simulink model "test14_r2019b"  (R2022b)
settings: Solver=VariableStepAuto  StartTime=0.0  StopTime=20  FixedStep=0.001  MaxStep=0.1  RelTol=1e-3
model workspace: external: MATLAB File E:\Hoc\do an\(final) download\test14_DataFile.m (data not in the file)
undefined symbols (not defined in the file): h, km, m, s, smiData, X, Y, Z
libraries: sm_lib x318, aerolibconvert2 x31, simulink_extras x25, nesl_utility x22, autolibshared x6, slpidlib x2, vehdynlibsteering x1
(part 1 of 9)
settings Model: Creator=ASUS  LastModifiedBy=ASUS
settings SolverCC: ZeroCrossAlgorithm=Adaptive  AlgebraicLoopSolver=LineSearch
settings DebuggingCC: IgnoredZcDiagnostic=none

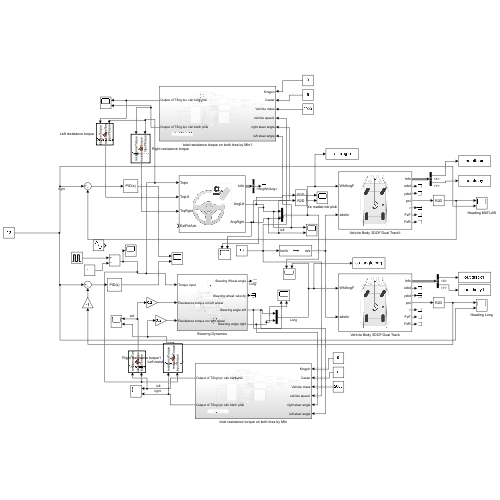
[thumbnail: Simulink's stored preview of the top-level diagram]
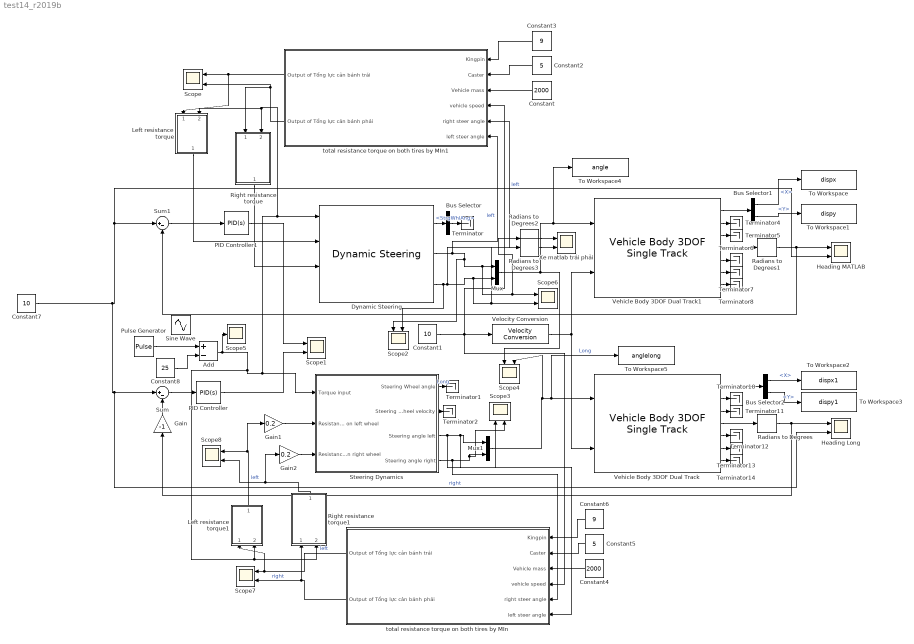
== system test14_r2019b ==
  Add : Sum  Inputs=+-
  Bus Selector : BusSelector  OutputSignals=StrgWhlAng
  Bus Selector1 : BusSelector  OutputSignals=InertFrm.Cg.Disp.X,InertFrm.Cg.Disp.Y
  Bus Selector2 : BusSelector  OutputSignals=InertFrm.Cg.Disp.X,InertFrm.Cg.Disp.Y
  Constant : Constant  Value=2000
  Constant1 : Constant  Value=10
  Constant2 : Constant  Value=5
  Constant3 : Constant  Value=9
  Constant4 : Constant  Value=2000
  Constant5 : Constant  Value=5
  Constant6 : Constant  Value=9
  Constant7 : Constant  Value=10
  Constant8 : Constant  Value=25
  Dynamic Steering : vehdynlibsteering/Dynamic Steering  StrgType=Rack and pinion  StrgRatioType=Constant  PwrAst=off  Loc=Front  TrckWdth=1  WhlBase=1.524  StrgRng=1.75*pi  StrgAngBpts="[-6.2832   -5.0265   -3.7699   -2.5133   -1.2566         0    1.2566    2.5133    3.7699    5.0265    6.2832]"  StrgRatioTbl=|  StrgRatio=13.5  StrgArmLngth=0.1  RckCsLngth=0.5  TieRodLngth=0.248  D=0.2  PnnRadiusTbl="[0.0055    0.0055    0.0056    0.0057    0.0057    0.0057    0.0058    0.0057    0.0056    0.0055    0.0055]"  PnnRadius=0.0057  RodLngth=0.1  ParaArmLngth=0.9  J1=0.1  J2=0.01  beta_u=0.1  beta_l=0.1  b1=0.001  k1=30  b2=1  b3=0.001  theta_o=0  omega_o=0  FricTrq=0  TrqBpts=[-100 0 100]  VehSpdBpts=[0 20]  TrqTbl=[0 -100;0 0;0 100]  TrqLmt=100  PwrLmt=1000  Eta=1  omega_c=200  aMode=2
      | [13.5000   13.3750   13.2500   13.1250   13.0000   13.0000   13.0000   13.1250   13.2500   13.3750   13.5000
      | ]
  Gain : Gain  Gain=-1
  Gain1 : Gain  Gain=0.2
  Gain2 : Gain  Gain=0.2
  Heading Long : Scope  NumInputPorts=2
  Heading MATLAB : Scope  NumInputPorts=2
  Left resistance torque : MATLAB Function  TreatAsAtomicUnit=on
  Left resistance torque1 : MATLAB Function  TreatAsAtomicUnit=on
  Mux : Mux  Inputs=2
  Mux1 : Mux  Inputs=2
  PID Controller : slpidlib/PID Controller  Controller=PID  Form=Parallel  TimeDomain=Continuous-time  UseExternalTs=off  SampleTime=-1  IntegratorMethod=Forward Euler  FilterMethod=Forward Euler  ControllerParametersSource=internal  P=1  I=1  UseKiTs=off  D=1  N=100  UseFilter=on  TunerSelectOption=Transfer Function Based (PID Tuner App)  InitialConditionSource=internal  InitialConditionForIntegrator=0  InitialConditionForFilter=0  DifferentiatorICPrevScaledInput=0  ExternalReset=none  TrackingMode=off  Kt=1  LimitOutput=off  SatLimitsSource=internal  UpperSaturationLimit=inf  LowerSaturationLimit=-inf  LinearizeAsGain=on  AntiWindupMode=none  Kb=1  LimitIntegrator=off  UpperIntegratorSaturationLimit=inf  LowerIntegratorSaturationLimit=-inf  POutMin=[]  POutMax=[]  IOutMin=[]  IOutMax=[]  DOutMin=[]  DOutMax=[]  NOutMin=[]  NOutMax=[]  SumOutMin=[]  SumOutMax=[]  SaturationOutMin=[]  SaturationOutMax=[]  PParamMin=[]  PParamMax=[]  IParamMin=[]  IParamMax=[]  DParamMin=[]  DParamMax=[]  NParamMin=[]  NParamMax=[]  KbParamMin=[]  KbParamMax=[]  KtParamMin=[]  KtParamMax=[]  KbOutMin=[]  KbOutMax=[]  KtOutMin=[]  KtOutMax=[]  IntegratorOutMin=[]  IntegratorOutMax=[]  FilterOutMin=[]  FilterOutMax=[]  SumI1OutMin=[]  SumI1OutMax=[]  SumI2OutMin=[]  SumI2OutMax=[]  SumI3OutMin=[]  SumI3OutMax=[]  SumI4OutMin=[]  SumI4OutMax=[]  SumDOutMin=[]  SumDOutMax=[]  DifferentiatorOutMin=[]  DifferentiatorOutMax=[]  FilterDiffOutCoefMin=[]  FilterDiffOutCoefMax=[]  ReciprocalOutMin=[]  ReciprocalOutMax=[]  SumDenOutMin=[]  SumDenOutMax=[]  SumNumOutMin=[]  SumNumOutMax=[]  DivideOutMin=[]  DivideOutMax=[]  UdiffTsProdOutMin=[]  UdiffTsProdOutMax=[]  NTsProdOutMin=[]  NTsProdOutMax=[]  UintegralTsProdOutMin=[]  UintegralTsProdOutMax=[]  UngainTsProdOutMin=[]  UngainTsProdOutMax=[]  ClampingZeroOutDataTypeStr=Inherit: Inherit via back propagation  ClampingZeroOutMin=[]  ClampingZeroOutMax=[]  FilterDenConstantOutDataTypeStr=Inherit: Inherit via back propagation  FilterDenConstantOutMin=[]  FilterDenConstantOutMax=[]  PCopyOutDataTypeStr=Inherit: Inherit via back propagation  PCopyOutMin=[]  PCopyOutMax=[]  NCopyOutDataTypeStr=Inherit: Inherit via back propagation  NCopyOutMin=[]  NCopyOutMax=[]  IntegratorContinuousStateAttributes=''  IntegratorStateMustResolveToSignalObject=off  IntegratorRTWStateStorageClass=Auto  FilterContinuousStateAttributes=''  FilterStateMustResolveToSignalObject=off  FilterRTWStateStorageClass=Auto  ParallelPVariant=InternalParameters  IdealPVariant=Disabled  IVariant=InternalParameters  DVariant=InternalParameters  IntegratorVariant=Continuous  SatVariant=Disabled  AWVariant=Passthrough  PCopyVariant=Disabled  TRVariant=Disabled  FdbkBlocksVariant=Forward  IdealPFdbkVariant=Disabled  SatFdbkVariant=Disabled  DerivativeFilterVariant=ContFilter  NVariant=InternalParameters  NCopyVariant=Disabled  FilterICVariant=InternalICsFilter  IntegratorICVariant=InternalICs  ExternalResetVariant=Disabled  TRSumVariant=Passthrough  SumFdbkVariant=Disabled  SumVariant=Sum_PID  TsampFilterVariant=InternalTs  TsampNgainVariant=Passthrough  TsampIntegralVariant=Passthrough  ExternalSaturationOutDataTypeStr=Inherit: Same as second input
  PID Controller1 : slpidlib/PID Controller  Controller=PID  Form=Parallel  TimeDomain=Continuous-time  UseExternalTs=off  SampleTime=-1  IntegratorMethod=Forward Euler  FilterMethod=Forward Euler  ControllerParametersSource=internal  P=1  I=1  UseKiTs=off  D=1  N=100  UseFilter=on  TunerSelectOption=Transfer Function Based (PID Tuner App)  InitialConditionSource=internal  InitialConditionForIntegrator=0  InitialConditionForFilter=0  DifferentiatorICPrevScaledInput=0  ExternalReset=none  TrackingMode=off  Kt=1  LimitOutput=off  SatLimitsSource=internal  UpperSaturationLimit=inf  LowerSaturationLimit=-inf  LinearizeAsGain=on  AntiWindupMode=none  Kb=1  LimitIntegrator=off  UpperIntegratorSaturationLimit=inf  LowerIntegratorSaturationLimit=-inf  POutMin=[]  POutMax=[]  IOutMin=[]  IOutMax=[]  DOutMin=[]  DOutMax=[]  NOutMin=[]  NOutMax=[]  SumOutMin=[]  SumOutMax=[]  SaturationOutMin=[]  SaturationOutMax=[]  PParamMin=[]  PParamMax=[]  IParamMin=[]  IParamMax=[]  DParamMin=[]  DParamMax=[]  NParamMin=[]  NParamMax=[]  KbParamMin=[]  KbParamMax=[]  KtParamMin=[]  KtParamMax=[]  KbOutMin=[]  KbOutMax=[]  KtOutMin=[]  KtOutMax=[]  IntegratorOutMin=[]  IntegratorOutMax=[]  FilterOutMin=[]  FilterOutMax=[]  SumI1OutMin=[]  SumI1OutMax=[]  SumI2OutMin=[]  SumI2OutMax=[]  SumI3OutMin=[]  SumI3OutMax=[]  SumI4OutMin=[]  SumI4OutMax=[]  SumDOutMin=[]  SumDOutMax=[]  DifferentiatorOutMin=[]  DifferentiatorOutMax=[]  FilterDiffOutCoefMin=[]  FilterDiffOutCoefMax=[]  ReciprocalOutMin=[]  ReciprocalOutMax=[]  SumDenOutMin=[]  SumDenOutMax=[]  SumNumOutMin=[]  SumNumOutMax=[]  DivideOutMin=[]  DivideOutMax=[]  UdiffTsProdOutMin=[]  UdiffTsProdOutMax=[]  NTsProdOutMin=[]  NTsProdOutMax=[]  UintegralTsProdOutMin=[]  UintegralTsProdOutMax=[]  UngainTsProdOutMin=[]  UngainTsProdOutMax=[]  ClampingZeroOutDataTypeStr=Inherit: Inherit via back propagation  ClampingZeroOutMin=[]  ClampingZeroOutMax=[]  FilterDenConstantOutDataTypeStr=Inherit: Inherit via back propagation  FilterDenConstantOutMin=[]  FilterDenConstantOutMax=[]  PCopyOutDataTypeStr=Inherit: Inherit via back propagation  PCopyOutMin=[]  PCopyOutMax=[]  NCopyOutDataTypeStr=Inherit: Inherit via back propagation  NCopyOutMin=[]  NCopyOutMax=[]  IntegratorContinuousStateAttributes=''  IntegratorStateMustResolveToSignalObject=off  IntegratorRTWStateStorageClass=Auto  FilterContinuousStateAttributes=''  FilterStateMustResolveToSignalObject=off  FilterRTWStateStorageClass=Auto  ParallelPVariant=InternalParameters  IdealPVariant=Disabled  IVariant=InternalParameters  DVariant=InternalParameters  IntegratorVariant=Continuous  SatVariant=Disabled  AWVariant=Passthrough  PCopyVariant=Disabled  TRVariant=Disabled  FdbkBlocksVariant=Forward  IdealPFdbkVariant=Disabled  SatFdbkVariant=Disabled  DerivativeFilterVariant=ContFilter  NVariant=InternalParameters  NCopyVariant=Disabled  FilterICVariant=InternalICsFilter  IntegratorICVariant=InternalICs  ExternalResetVariant=Disabled  TRSumVariant=Passthrough  SumFdbkVariant=Disabled  SumVariant=Sum_PID  TsampFilterVariant=InternalTs  TsampNgainVariant=Passthrough  TsampIntegralVariant=Passthrough  ExternalSaturationOutDataTypeStr=Inherit: Same as second input
  Pulse Generator : DiscretePulseGenerator  PulseType=Time based  Amplitude=50  Period=10  PulseWidth=50
  Radians to Degrees{,1..3} (4 alike) : simulink_extras/Transformations/Radians to Degrees
  Right resistance torque : MATLAB Function  TreatAsAtomicUnit=on
  Right resistance torque1 : MATLAB Function  TreatAsAtomicUnit=on
  Scope{,1..4,6..8} (8 alike) : Scope  NumInputPorts=2
  Scope5 : Scope
  Sine Wave : Sin  Amplitude=80  Frequency=3  SampleTime=0
  Steering Dynamics : Subsystem
  Sum : Sum  Inputs=|+-
  Sum1 : Sum  Inputs=|+-
  Terminator{,1..2,4..8,10..14} (13 alike) : Terminator
  To Workspace : ToWorkspace  VariableName=dispx  SaveFormat=Structure With Time  SampleTime=-1
  To Workspace1 : ToWorkspace  VariableName=dispy  SaveFormat=Structure With Time  SampleTime=-1
  To Workspace2 : ToWorkspace  VariableName=dispx1  SaveFormat=Structure With Time  SampleTime=-1
  To Workspace3 : ToWorkspace  VariableName=dispy1  SaveFormat=Structure With Time  SampleTime=-1
  To Workspace4 : ToWorkspace  VariableName=angle  SaveFormat=Structure With Time  SampleTime=-1
  To Workspace5 : ToWorkspace  VariableName=anglelong  SaveFormat=Structure With Time  SampleTime=-1
  Vehicle Body 3DOF Dual Track : autolibshared/Vehicle Body 3DOF Single Track  trackMode=Dual  inputMode=External longitudinal velocity  frontSteerMode=on  rearSteerMode=off  windMode=off  muMode=off  extFMode=off  extMMode=off  htchFMode=off  htchMMode=off  extXo=off  extpsio=off  extxdoto=off  extro=off  extYo=off  extTamb=off  extydoto=off  aMode=2  NF=2  NR=2  m=2000  a=1.4  b=1.6  h=0.35  dh=1  hh=0.2  X_o=0  xdot_o=0  CalphaMode=off  sigmaMode=on  d=0  hl=0  w=[1.4,1.4]  Cy_f=12e3  Cy_r=11e3  sigma_f=.1  sigma_r=.1  alpha_f_brk=[-.1 .1]  Cy_f_data=[-9e3 9e3]  alpha_r_brk=[-.1 .1]  Cy_r_data=[-9e3 9e3]  Y_o=0  ydot_o=0  Izz=4000  psi_o=0  r_o=0  Af=2  Cd=.3  Cl=.1  Cpm=.1  beta_w=[0:0.01:0.3]  Cs=[0:0.03:0.9]  Cym=[0:0.01:0.3]  Pabs=101325  Tair=273  g=9.81  mu=1  xdot_tol=.01  Fznom=5000  Fxtire_sat=7e4  Fytire_sat=7e4  longOff=0  latOff=0  vertOff=0  wrapAng=off
  Vehicle Body 3DOF Dual Track1 : autolibshared/Vehicle Body 3DOF Single Track  trackMode=Dual  inputMode=External longitudinal velocity  frontSteerMode=on  rearSteerMode=off  windMode=off  muMode=off  extFMode=off  extMMode=off  htchFMode=off  htchMMode=off  extXo=off  extpsio=off  extxdoto=off  extro=off  extYo=off  extTamb=off  extydoto=off  aMode=2  NF=2  NR=2  m=2000  a=1.4  b=1.6  h=0.35  dh=1  hh=0.2  X_o=0  xdot_o=0  CalphaMode=off  sigmaMode=on  d=0  hl=0  w=[1.4,1.4]  Cy_f=12e3  Cy_r=11e3  sigma_f=.1  sigma_r=.1  alpha_f_brk=[-.1 .1]  Cy_f_data=[-9e3 9e3]  alpha_r_brk=[-.1 .1]  Cy_r_data=[-9e3 9e3]  Y_o=0  ydot_o=0  Izz=4000  psi_o=0  r_o=0  Af=2  Cd=.3  Cl=.1  Cpm=.1  beta_w=[0:0.01:0.3]  Cs=[0:0.03:0.9]  Cym=[0:0.01:0.3]  Pabs=101325  Tair=273  g=9.81  mu=1  xdot_tol=.01  Fznom=5000  Fxtire_sat=7e4  Fytire_sat=7e4  longOff=0  latOff=0  vertOff=0  wrapAng=off
  Velocity Conversion : aerolibconvert2/Velocity Conversion  IU=km/h  OU=m/s
  Xe matlab trái phải : Scope  NumInputPorts=2
  total resistance torque on both tires by MIn : Subsystem
  total resistance torque on both tires by MIn1 : Subsystem
  wires:
  Dynamic Steering/2 -> total resistance torque on both tires by MIn1/6(left steer angle), Scope2/1, Radians to Degrees2/1, Scope6/1, Mux/1  "left"
  Dynamic Steering/3 -> Scope2/2, total resistance torque on both tires by MIn1/5(right steer angle), Radians to Degrees3/1, Scope6/2, Mux/2  "left"
  Steering Dynamics/3(Steering angle left) -> Scope3/1, total resistance torque on both tires by MIn/6(left steer angle), Mux1/1
  Steering Dynamics/4(Steering angle right) -> total resistance torque on both tires by MIn/5(right steer angle), Scope3/2, Mux1/2
  Mux1/1 -> Vehicle Body 3DOF Dual Track/1, To Workspace5/1, Scope4/2  "Long"
  Velocity Conversion/1 -> Vehicle Body 3DOF Dual Track/2, Vehicle Body 3DOF Dual Track1/2
  Constant1/1 -> total resistance torque on both tires by MIn1/4("vehicle speed "), total resistance torque on both tires by MIn/4("vehicle speed "), Velocity Conversion/1
  Vehicle Body 3DOF Dual Track1/4 -> Radians to Degrees1/1
  Vehicle Body 3DOF Dual Track/4 -> Radians to Degrees/1
  Radians to Degrees/1 -> Heading Long/1, Gain/1
  Steering Dynamics/2(Steering wheel velocity) -> Terminator2/1
  Vehicle Body 3DOF Dual Track1/1 -> Bus Selector1/1
  Vehicle Body 3DOF Dual Track1/2 -> Terminator4/1
  Vehicle Body 3DOF Dual Track1/3 -> Terminator5/1
  Vehicle Body 3DOF Dual Track1/5 -> Terminator6/1
  Vehicle Body 3DOF Dual Track1/6 -> Terminator7/1
  Vehicle Body 3DOF Dual Track1/7 -> Terminator8/1
  Vehicle Body 3DOF Dual Track/2 -> Terminator10/1
  Vehicle Body 3DOF Dual Track/3 -> Terminator11/1
  Vehicle Body 3DOF Dual Track/5 -> Terminator12/1
  Vehicle Body 3DOF Dual Track/6 -> Terminator13/1
  Vehicle Body 3DOF Dual Track/7 -> Terminator14/1
  Dynamic Steering/1 -> Bus Selector/1
  Bus Selector/1 -> Terminator/1  "<StrgWhlAng>"
  Bus Selector1/1 -> To Workspace/1  "<X>"
  Bus Selector1/2 -> To Workspace1/1  "<Y>"
  total resistance torque on both tires by MIn1/2(Output of Tổng lực cản bánh phải) -> Scope/2, Right resistance torque/1("resistanceTorque ")
  Constant/1 -> total resistance torque on both tires by MIn1/3(Vehicle mass)
  Constant2/1 -> total resistance torque on both tires by MIn1/2(Caster)
  Constant3/1 -> total resistance torque on both tires by MIn1/1(Kingpin)
  Constant4/1 -> total resistance torque on both tires by MIn/3(Vehicle mass)
  Constant5/1 -> total resistance torque on both tires by MIn/2(Caster)
  Constant6/1 -> total resistance torque on both tires by MIn/1(Kingpin)
  Vehicle Body 3DOF Dual Track/1 -> Bus Selector2/1
  Bus Selector2/1 -> To Workspace2/1  "<X>"
  Bus Selector2/2 -> To Workspace3/1  "<Y>"
  Steering Dynamics/1(Steering Wheel angle) -> Terminator1/1  "Long"
  Sum/1 -> PID Controller/1
  Sum1/1 -> PID Controller1/1
  PID Controller1/1 -> Scope1/1
  Radians to Degrees1/1 -> Sum1/2, Heading MATLAB/1
  PID Controller/1 -> Scope1/2
  Constant7/1 -> Heading Long/2, Sum/1, Heading MATLAB/2, Sum1/1  "right"
  Gain/1 -> Sum/2
  Mux/1 -> Scope4/1, To Workspace4/1, Vehicle Body 3DOF Dual Track1/1
  Pulse Generator/1 -> Add/1
  Constant8/1 -> Add/2
  total resistance torque on both tires by MIn/1(Output of Tổng lực cản bánh trái) -> Left resistance torque1/1("resistanceTorque "), Scope7/1  "left"
  total resistance torque on both tires by MIn/2(Output of Tổng lực cản bánh phải) -> Scope7/2, Right resistance torque1/1("resistanceTorque ")  "right"
  total resistance torque on both tires by MIn1/1(Output of Tổng lực cản bánh trái) -> Left resistance torque/1("resistanceTorque "), Scope/1
  Add/1 -> Scope5/1, Right resistance torque1/2(inputTorque), Left resistance torque1/2(inputTorque), Left resistance torque/2(inputTorque), Right resistance torque/2(inputTorque), Dynamic Steering/1, Steering Dynamics/1(Torque input)
  Left resistance torque1/1(resistanceTorque) -> Gain1/1, Scope8/1  "left"
  Radians to Degrees2/1 -> Xe matlab trái phải/1
  Radians to Degrees3/1 -> Xe matlab trái phải/2
  Right resistance torque1/1(resistanceTorque) -> Gain2/1, Scope8/2
  Right resistance torque/1(resistanceTorque) -> Dynamic Steering/3
  Left resistance torque/1(resistanceTorque) -> Dynamic Steering/2
  Gain1/1 -> Steering Dynamics/2(Resistance torque on left wheel)
  Gain2/1 -> Steering Dynamics/3(Resistance torque on right wheel)

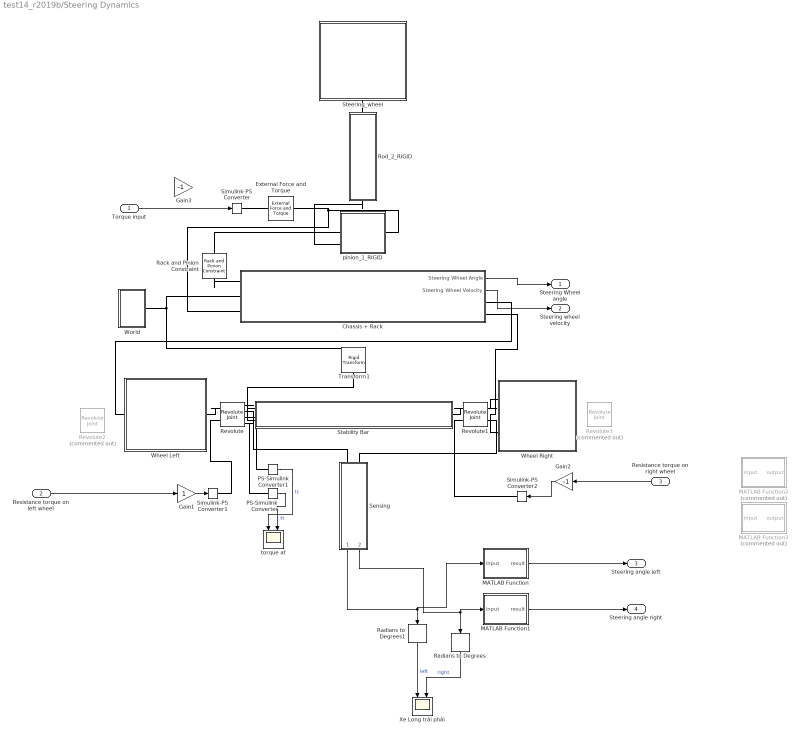
== system test14_r2019b/Steering Dynamics ==
  Torque input : Inport
  Resistance torque on left wheel : Inport  Port=2
  Resistance torque on right wheel : Inport  Port=3
  Chassis + Rack : Subsystem
      mask Display: image('$imagefile'); % Use "Edit Image" on toolstrip to change.
  External Force and Torque : sm_lib/Forces and Torques/External Force and Torque  ForceResolutionFrame=AttachedFrame  EnableForceX=off  EnableForceY=off  EnableForceZ=off  EnableForce=off  TorqueResolutionFrame=AttachedFrame  EnableTorqueX=off  EnableTorqueY=off  EnableTorqueZ=on  EnableTorque=off
  Gain1 : Gain
  Gain2 : Gain  Gain=-1
  Gain3 : Gain  Gain=-1
  MATLAB Function : MATLAB Function  TreatAsAtomicUnit=on
  MATLAB Function1 : MATLAB Function  TreatAsAtomicUnit=on
  MATLAB Function2 : MATLAB Function  Commented=on  TreatAsAtomicUnit=on
  MATLAB Function3 : MATLAB Function  Commented=on  TreatAsAtomicUnit=on
  PS-Simulink Converter : nesl_utility/PS-Simulink Converter  PhysicalDomain=network_engine_domain  SubClassName=ps_output  LeftPortType=input  RightPortType=output  PseudoPeriodic=off  Frequencies=[]  VectorFormat=inherit  Unit=inherit  AffineConversion=off
  PS-Simulink Converter1 : nesl_utility/PS-Simulink Converter  PhysicalDomain=network_engine_domain  SubClassName=ps_output  LeftPortType=input  RightPortType=output  PseudoPeriodic=off  Frequencies=[]  VectorFormat=inherit  Unit=inherit  AffineConversion=off
  Rack and Pinion Constraint : sm_lib/Gears and Couplings/Gears/Rack and Pinion Constraint  PinionRadius=30  PinionRadiusUnits=mm
  Radians to Degrees : simulink_extras/Transformations/Radians to Degrees
  Radians to Degrees1 : simulink_extras/Transformations/Radians to Degrees
  Revolute : sm_lib/Joints/Revolute Joint  JointMode=Normal  SenseConstraintForce=off  SenseConstraintForceX=off  SenseConstraintForceY=off  SenseConstraintForceZ=off  SenseConstraintTorque=on  SenseConstraintTorqueX=off  SenseConstraintTorqueY=off  SenseConstraintTorqueZ=off  SenseTotalForce=off  SenseTotalForceX=off  SenseTotalForceY=off  SenseTotalForceZ=off  SenseTotalTorque=on  SenseTotalTorqueX=off  SenseTotalTorqueY=off  SenseTotalTorqueZ=off  CompositeWrenchDir=BaseOnFollower  CompositeWrenchFrame=FollowerFrame  EquilibriumPosition=0  EquilibriumPositionUnits=deg  SpringStiffness=0.0524-0.0524+0.1  SpringStiffnessUnits=N*m/deg  DampingCoefficient=1.5-1.5+0.1  DampingCoefficientUnits=N*m/(deg/s)  TorqueActuationMode=InputTorque  MotionActuationMode=ComputedMotion  SensePosition=on  SenseVelocity=off  SenseAcceleration=off  SenseTorqueForce=off  SenseLowerLimitTorqueForce=off  SenseUpperLimitTorqueForce=off  LowerLimitSpecify=on  LowerLimitBound=-89.68-28.95  LowerLimitBoundUnits=deg  LowerLimitStiffness=1e4  LowerLimitStiffnessUnits=N*m/deg  LowerLimitDamping=100  LowerLimitDampingUnits=N*m/(deg/s)  LowerLimitTransitionRegionWidth=0.1  LowerLimitTransitionRegionWidthUnits=deg  UpperLimitSpecify=on  UpperLimitBound=-89.68+18.80  UpperLimitBoundUnits=deg  UpperLimitStiffness=1e4  UpperLimitStiffnessUnits=N*m/deg  UpperLimitDamping=100  UpperLimitDampingUnits=N*m/(deg/s)  UpperLimitTransitionRegionWidth=0.1  UpperLimitTransitionRegionWidthUnits=deg  PositionTargetSpecify=on  PositionTargetPriority=High  PositionTargetValue=-89.678329494  PositionTargetValueUnits=deg  VelocityTargetSpecify=on  VelocityTargetPriority=High  VelocityTargetValue=0  VelocityTargetValueUnits=deg/s
  Revolute1 : sm_lib/Joints/Revolute Joint  JointMode=Normal  SenseConstraintForce=off  SenseConstraintForceX=off  SenseConstraintForceY=off  SenseConstraintForceZ=off  SenseConstraintTorque=off  SenseConstraintTorqueX=off  SenseConstraintTorqueY=off  SenseConstraintTorqueZ=off  SenseTotalForce=off  SenseTotalForceX=off  SenseTotalForceY=off  SenseTotalForceZ=off  SenseTotalTorque=off  SenseTotalTorqueX=off  SenseTotalTorqueY=off  SenseTotalTorqueZ=off  CompositeWrenchDir=FollowerOnBase  CompositeWrenchFrame=FollowerFrame  EquilibriumPosition=0  EquilibriumPositionUnits=deg  SpringStiffness=0.1  SpringStiffnessUnits=N*m/deg  DampingCoefficient=0.1  DampingCoefficientUnits=N*m/(deg/s)  TorqueActuationMode=InputTorque  MotionActuationMode=ComputedMotion  SensePosition=on  SenseVelocity=off  SenseAcceleration=off  SenseTorqueForce=off  SenseLowerLimitTorqueForce=off  SenseUpperLimitTorqueForce=off  LowerLimitSpecify=on  LowerLimitBound=-89.68-28.95  LowerLimitBoundUnits=deg  LowerLimitStiffness=1e4  LowerLimitStiffnessUnits=N*m/deg  LowerLimitDamping=100  LowerLimitDampingUnits=N*m/(deg/s)  LowerLimitTransitionRegionWidth=0.1  LowerLimitTransitionRegionWidthUnits=deg  UpperLimitSpecify=on  UpperLimitBound=-89.68+18.80  UpperLimitBoundUnits=deg  UpperLimitStiffness=1e4  UpperLimitStiffnessUnits=N*m/deg  UpperLimitDamping=100  UpperLimitDampingUnits=N*m/(deg/s)  UpperLimitTransitionRegionWidth=0.1  UpperLimitTransitionRegionWidthUnits=deg  PositionTargetSpecify=on  PositionTargetPriority=Low  PositionTargetValue=smiData.RevoluteJoint(2).Rz.Pos-2.7  PositionTargetValueUnits=deg  VelocityTargetSpecify=on  VelocityTargetPriority=High  VelocityTargetValue=0  VelocityTargetValueUnits=deg/s
  Revolute2 : sm_lib/Joints/Revolute Joint  Commented=on  JointMode=Normal  SenseConstraintForce=off  SenseConstraintForceX=off  SenseConstraintForceY=off  SenseConstraintForceZ=off  SenseConstraintTorque=off  SenseConstraintTorqueX=off  SenseConstraintTorqueY=off  SenseConstraintTorqueZ=off  SenseTotalForce=off  SenseTotalForceX=off  SenseTotalForceY=off  SenseTotalForceZ=off  SenseTotalTorque=off  SenseTotalTorqueX=off  SenseTotalTorqueY=off  SenseTotalTorqueZ=off  CompositeWrenchDir=BaseOnFollower  CompositeWrenchFrame=FollowerFrame  EquilibriumPosition=0  EquilibriumPositionUnits=deg  SpringStiffness=0.0524-0.0524+0.1  SpringStiffnessUnits=N*m/deg  DampingCoefficient=1.5-1.5+0.1  DampingCoefficientUnits=N*m/(deg/s)  TorqueActuationMode=InputTorque  MotionActuationMode=ComputedMotion  SensePosition=on  SenseVelocity=off  SenseAcceleration=off  SenseTorqueForce=off  SenseLowerLimitTorqueForce=off  SenseUpperLimitTorqueForce=off  LowerLimitSpecify=on  LowerLimitBound=-2+0.089+0.071  LowerLimitBoundUnits=rad  LowerLimitStiffness=1e4  LowerLimitStiffnessUnits=N*m/deg  LowerLimitDamping=100  LowerLimitDampingUnits=N*m/(deg/s)  LowerLimitTransitionRegionWidth=0.1  LowerLimitTransitionRegionWidthUnits=deg  UpperLimitSpecify=on  UpperLimitBound=-1-0.195-0.106  UpperLimitBoundUnits=rad  UpperLimitStiffness=1e4  UpperLimitStiffnessUnits=N*m/deg  UpperLimitDamping=100  UpperLimitDampingUnits=N*m/(deg/s)  UpperLimitTransitionRegionWidth=0.1  UpperLimitTransitionRegionWidthUnits=deg  PositionTargetSpecify=on  PositionTargetPriority=High  PositionTargetValue=-89.678329494  PositionTargetValueUnits=deg  VelocityTargetSpecify=on  VelocityTargetPriority=High  VelocityTargetValue=0  VelocityTargetValueUnits=deg/s
  Revolute3 : sm_lib/Joints/Revolute Joint  Commented=on  JointMode=Normal  SenseConstraintForce=off  SenseConstraintForceX=off  SenseConstraintForceY=off  SenseConstraintForceZ=off  SenseConstraintTorque=off  SenseConstraintTorqueX=off  SenseConstraintTorqueY=off  SenseConstraintTorqueZ=off  SenseTotalForce=off  SenseTotalForceX=off  SenseTotalForceY=off  SenseTotalForceZ=off  SenseTotalTorque=off  SenseTotalTorqueX=off  SenseTotalTorqueY=off  SenseTotalTorqueZ=off  CompositeWrenchDir=FollowerOnBase  CompositeWrenchFrame=FollowerFrame  EquilibriumPosition=0  EquilibriumPositionUnits=deg  SpringStiffness=0.1  SpringStiffnessUnits=N*m/deg  DampingCoefficient=0.1  DampingCoefficientUnits=N*m/(deg/s)  TorqueActuationMode=InputTorque  MotionActuationMode=ComputedMotion  SensePosition=on  SenseVelocity=off  SenseAcceleration=off  SenseTorqueForce=off  SenseLowerLimitTorqueForce=off  SenseUpperLimitTorqueForce=off  LowerLimitSpecify=off  LowerLimitBound=-2  LowerLimitBoundUnits=rad  LowerLimitStiffness=1e4  LowerLimitStiffnessUnits=N*m/deg  LowerLimitDamping=100  LowerLimitDampingUnits=N*m/(deg/s)  LowerLimitTransitionRegionWidth=0.1  LowerLimitTransitionRegionWidthUnits=deg  UpperLimitSpecify=off  UpperLimitBound=-1  UpperLimitBoundUnits=rad  UpperLimitStiffness=1e4  UpperLimitStiffnessUnits=N*m/deg  UpperLimitDamping=100  UpperLimitDampingUnits=N*m/(deg/s)  UpperLimitTransitionRegionWidth=0.1  UpperLimitTransitionRegionWidthUnits=deg  PositionTargetSpecify=on  PositionTargetPriority=Low  PositionTargetValue=smiData.RevoluteJoint(2).Rz.Pos-2.7  PositionTargetValueUnits=deg  VelocityTargetSpecify=on  VelocityTargetPriority=High  VelocityTargetValue=0  VelocityTargetValueUnits=deg/s
  Rod_2_RIGID : Subsystem
      mask Display: image('rod.png'); % Use "Edit Image" on toolstrip to change.
  "Sensing " : Subsystem
  Simulink-PS Converter : nesl_utility/Simulink-PS Converter  PhysicalDomain=network_engine_domain  SubClassName=ps_input  LeftPortType=input  RightPortType=output  PseudoPeriodic=off  Frequencies=[]  NoiseDistribution=none  NoiseParameters=[]  Unit=N*m  AffineConversion=off  FilteringAndDerivatives=provide  SimscapeFilterOrder=1  InputFilterTimeConstant=0.001  UdotUserProvided=0
  Simulink-PS Converter1 : nesl_utility/Simulink-PS Converter  PhysicalDomain=network_engine_domain  SubClassName=ps_input  LeftPortType=input  RightPortType=output  PseudoPeriodic=off  Frequencies=[]  NoiseDistribution=none  NoiseParameters=[]  Unit=N*m  AffineConversion=off  FilteringAndDerivatives=provide  SimscapeFilterOrder=1  InputFilterTimeConstant=0.001  UdotUserProvided=0
  Simulink-PS Converter2 : nesl_utility/Simulink-PS Converter  PhysicalDomain=network_engine_domain  SubClassName=ps_input  LeftPortType=input  RightPortType=output  PseudoPeriodic=off  Frequencies=[]  NoiseDistribution=none  NoiseParameters=[]  Unit=N*m  AffineConversion=off  FilteringAndDerivatives=provide  SimscapeFilterOrder=2  InputFilterTimeConstant=0.001  UdotUserProvided=0
  Stability Bar : Subsystem
      mask Display: image('$imagefile'); % Use "Edit Image" on toolstrip to change.
  Steering_wheel : Subsystem
      mask Display: image('$imagefile'); % Use "Edit Image" on toolstrip to change.
  Transform1 : sm_lib/Frames and Transforms/Rigid Transform  TranslationMethod=Cartesian  TranslationStandardOffset=0  TranslationLengthUnit=mm  TranslationStandardAxis=+Z  TranslationCartesianOffset=smiData.RigidTransform(48).translation  TranslationROffset=0  TranslationROffsetUnits=m  TranslationZOffset=0  TranslationZOffsetUnits=m  TranslationThetaOffset=0  TranslationThetaOffsetUnits=deg  RotationMethod=ArbitraryAxis  RotationAngleUnits=rad  RotationStandardAxis=+Z  RotationAngle=smiData.RigidTransform(48).angle  RotationArbitraryAxis=smiData.RigidTransform(48).axis  FollAlignAxisA=+X  BaseAlignAxisA=+Y  FollAlignAxisB=+Y  BaseAlignAxisB=+Z  RotationSequenceAxes=FollowerAxes  RotationSequence=XYX  RotationSequenceAngles=[0 0 0]  RotationSequenceAnglesUnits=deg  RotationMatrix=[1 0 0; 0 1 0; 0 0 1]  Quaternion=[1 0 0 0]
  Wheel Left : Subsystem
      mask Display: image('$imagefile'); % Use "Edit Image" on toolstrip to change.
  Wheel Right : Subsystem
      mask Display: image('$imagefile'); % Use "Edit Image" on toolstrip to change.
  World : Subsystem
  Xe Long trái phải : Scope  NumInputPorts=2
  pinion_1_RIGID : Subsystem
      mask Display: image('pinion.png'); % Use "Edit Image" on toolstrip to change.
  "torque at " : Scope  NumInputPorts=2
  Steering Wheel angle : Outport
  Steering wheel velocity : Outport  Port=2
  Steering angle left : Outport  Port=3
  Steering angle right : Outport  Port=4
  wires:
  "Sensing "/2(Steering angle right (rad)) -> MATLAB Function1/1(input), Radians to Degrees/1
  Radians to Degrees/1 -> Xe Long trái phải/2  "right"
  Radians to Degrees1/1 -> Xe Long trái phải/1  "left"
  Chassis + Rack/2(Steering Wheel Velocity) -> Steering wheel velocity/1
  Chassis + Rack/1(Steering Wheel Angle) -> Steering Wheel angle/1
  Resistance torque on left wheel/1 -> Gain1/1
  Resistance torque on right wheel/1 -> Gain2/1
  Gain1/1 -> Simulink-PS Converter1/1
  Gain2/1 -> Simulink-PS Converter2/1
  MATLAB Function/1(result) -> Steering angle left/1
  MATLAB Function1/1(result) -> Steering angle right/1
  Torque input/1 -> Simulink-PS Converter/1
  "Sensing "/1(Steering angle left (rad)) -> MATLAB Function/1(input), Radians to Degrees1/1
  PS-Simulink Converter1/1 -> "torque at "/1  "tc"
  PS-Simulink Converter/1 -> "torque at "/2  "tt"
  connections:
  Revolute/RConn2 -- "Sensing "/LConn1
  Simulink-PS Converter/RConn1 -- External Force and Torque/LConn1
  Chassis + Rack/LConn2 -- World/LConn1 -- Transform1/LConn1
  Rack and Pinion Constraint/RConn1 -- Chassis + Rack/LConn1
  Revolute1/RConn2 -- "Sensing "/LConn2
  Rack and Pinion Constraint/LConn1 -- pinion_1_RIGID/LConn2
  Transform1/RConn1 -- Stability Bar/LConn2
  Chassis + Rack/LConn3 -- pinion_1_RIGID/RConn1 -- External Force and Torque/RConn1
  Chassis + Rack/RConn1 -- Wheel Left/LConn1
  Revolute1/RConn1 -- Wheel Right/LConn1
  Chassis + Rack/RConn2 -- Wheel Right/LConn2
  Revolute1/LConn1 -- Stability Bar/RConn1
  Revolute/RConn1 -- Stability Bar/LConn1
  Revolute/LConn1 -- Wheel Left/RConn1
  Rod_2_RIGID/RConn1 -- pinion_1_RIGID/LConn3
  Steering_wheel/LConn1 -- Rod_2_RIGID/LConn1
  Simulink-PS Converter1/RConn1 -- Revolute/LConn2
  Revolute1/LConn2 -- Simulink-PS Converter2/RConn1
  Revolute/RConn3 -- PS-Simulink Converter1/LConn1
  Revolute/RConn4 -- PS-Simulink Converter/LConn1

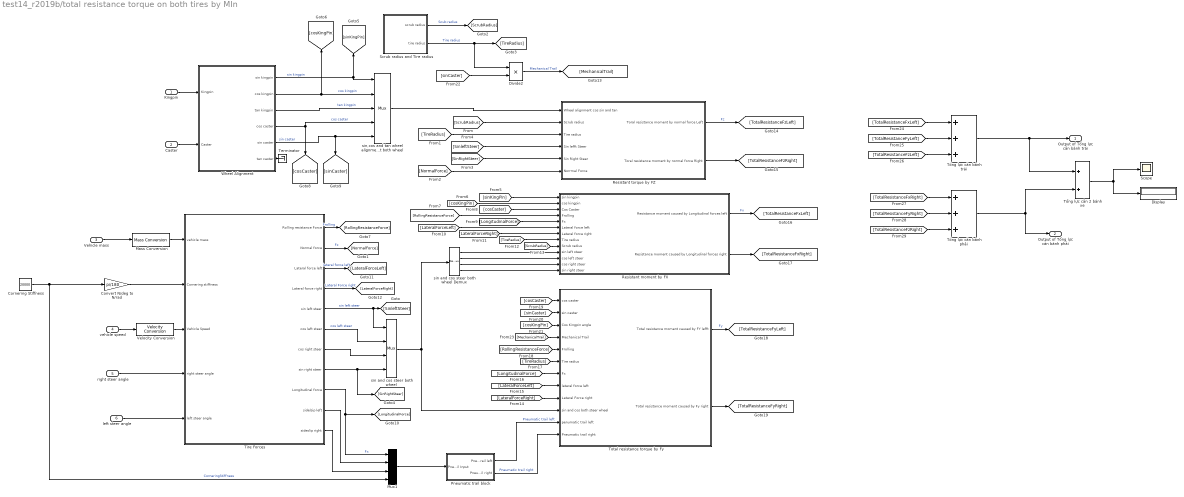
== system test14_r2019b/total resistance torque on both tires by MIn ==
  Kingpin : Inport
  Caster : Inport  Port=2
  Vehicle mass : Inport  Port=3
  "vehicle speed " : Inport  Port=4
  right steer angle : Inport  Port=5
  left steer angle : Inport  Port=6
  Convert N/deg to N/rad : Gain  Gain=pi/180
  Cornering Stiffness : Constant  Value=20000
  Display : Display
  Divide2 : Product  Inputs=**
  Mass Conversion : aerolibconvert2/Mass Conversion  IU=kg  OU=kg
  Mux1 : Mux
  Pneumatic trail block : Subsystem
  Resistant moment by FX : Subsystem
  Resistant torque by FZ : Subsystem
  Scope : Scope
  Scrub radius and Tire radius : Subsystem
  Terminator : Terminator
  Tire Forces : Subsystem
  Total resistance torque by Fy : Subsystem
  Tổng lực cản 2 bánh xe : Sum
  Tổng lực cản bánh phải : Sum  Inputs=+++
  Tổng lực cản bánh trái : Sum  Inputs=+++
  Velocity Conversion : aerolibconvert2/Velocity Conversion  IU=km/h  OU=m/s
  Wheel Alignment : Subsystem
  sin and cos steer both wheel : Mux
  sin and cos steer both wheel Demux : Demux
  sin,cos and tan wheel alignment both wheel : Mux  Inputs=5
  Output of Tổng lực cản bánh trái : Outport
  Output of Tổng lực cản bánh phải : Outport  Port=2
  wires:
  Kingpin/1 -> Wheel Alignment/1(Kingpin)
  Wheel Alignment/6(tan caster) -> Terminator/1
  Vehicle mass/1 -> Mass Conversion/1
  Mass Conversion/1 -> Tire Forces/1(vehicle mass)
  Convert N/deg to N/rad/1 -> Tire Forces/2(Cornering stiffness)
  Cornering Stiffness/1 -> Mux1/4, Convert N/deg to N/rad/1  "CorneringStiffness"
  Caster/1 -> Wheel Alignment/2(Caster)
  "vehicle speed "/1 -> Velocity Conversion/1
  right steer angle/1 -> Tire Forces/4("right steer angle ")
  left steer angle/1 -> Tire Forces/5("left steer angle ")
  Velocity Conversion/1 -> Tire Forces/3(Vehicle Speed)
  Tire Forces/11(sideslip right) -> Mux1/3
  Tire Forces/10(sidelsip left) -> Mux1/2
  Tire Forces/9(Longitudinal force) -> [LongitudinalForce], Mux1/1  "Fx"
  Mux1/1 -> Pneumatic trail block/1(Pneumatic trail Input)
  Pneumatic trail block/2(Pneumatic Trail right) -> Total resistance torque by Fy/12(Pneumatic trail right)  "Pneumatic trail right"
  Pneumatic trail block/1(Pneumatic Trail left) -> Total resistance torque by Fy/11(penumatic trail left)  "Pneumatic trail left"
  Tire Forces/5(sin left steer) -> sin and cos steer both wheel/1, [SinleftSteer]  "sin left steer"
  Tire Forces/6(cos left steer) -> sin and cos steer both wheel/2  "cos left steer"
  Tire Forces/7(cos right steer) -> sin and cos steer both wheel/3
  Tire Forces/8(sin right steer) -> [SinRightSteer], sin and cos steer both wheel/4
  sin and cos steer both wheel/1 -> sin and cos steer both wheel Demux/1, Total resistance torque by Fy/10(sin and cos both steer wheel)
  Wheel Alignment/1(sin kingpin) -> sin,cos and tan wheel alignment both wheel/1, [sinKingPin]  "sin kingpin"
  Wheel Alignment/2(cos kingpin) -> [cosKingPin], sin,cos and tan wheel alignment both wheel/2  "cos kingpin"
  Wheel Alignment/3(tan kingpin) -> sin,cos and tan wheel alignment both wheel/3  "tan kingpin"
  Wheel Alignment/4(cos caster) -> sin,cos and tan wheel alignment both wheel/4, [cosCaster]  "cos caster"
  Wheel Alignment/5(sin caster) -> [sinCaster], sin,cos and tan wheel alignment both wheel/5  "sin caster"
  sin,cos and tan wheel alignment both wheel/1 -> Resistant torque by FZ/1("Wheel alignment cos sin and tan ")
  Tire Forces/2(Normal force) -> [NormalForce]  "Fz"
  Scrub radius and Tire radius/1(scrub radius) -> [ScrubRadius]  "Scub radius"
  Scrub radius and Tire radius/2(tire radius) -> Divide2/1, [TireRadius]  "Tire radius"
  [ScrubRadius] -> Resistant torque by FZ/2(Scrub radius)
  [TireRadius] -> Resistant torque by FZ/3(Tire radius)
  [NormalForce] -> Resistant torque by FZ/6(Norrmal Force)
  [SinleftSteer] -> Resistant torque by FZ/4(Sin lefft Steer)
  [SinRightSteer] -> Resistant torque by FZ/5(Sin Right Steer)
  [sinKingPin] -> Resistant moment by FX/1(sin kingpin)
  [cosKingPin] -> Resistant moment by FX/2(cos kingpin)
  Tire Forces/1(Rolling resistance Force) -> [RollingResistanceForce]  "Frolling"
  [RollingResistanceForce] -> Resistant moment by FX/4(Frolling)
  [cosCaster] -> Resistant moment by FX/3(Cos Caster)
  [LongitudinalForce] -> Resistant moment by FX/5(Fx)
  Tire Forces/3(Lateral force left) -> [LateralForceLeft]  "lateral force left"
  Tire Forces/4(Lateral force right) -> [LateralForceRight]  "Lateral Force right"
  [LateralForceLeft] -> Resistant moment by FX/6(Lateral force left)
  [LateralForceRight] -> Resistant moment by FX/7(Lateral force right)
  [TireRadius] -> Resistant moment by FX/8(Tire radius)
  [ScrubRadius] -> Resistant moment by FX/9(Scrub radius)
  [LateralForceRight] -> Total resistance torque by Fy/9(Lateral Force right)
  [LateralForceLeft] -> Total resistance torque by Fy/8(lateral force left)
  [LongitudinalForce] -> Total resistance torque by Fy/7(Fx)
  [TireRadius] -> Total resistance torque by Fy/6(Tire radius)
  [RollingResistanceForce] -> Total resistance torque by Fy/5(Frolling)
  [sinCaster] -> Total resistance torque by Fy/2(sin caster)
  [cosCaster] -> Total resistance torque by Fy/1(cos caster)
  [cosKingPin] -> Total resistance torque by Fy/3(Cos Kingpin angle)
  sin and cos steer both wheel Demux/1 -> Resistant moment by FX/10(sin left steer)
  sin and cos steer both wheel Demux/2 -> Resistant moment by FX/11(cos left steer)
  sin and cos steer both wheel Demux/3 -> Resistant moment by FX/12(cos right steer)
  sin and cos steer both wheel Demux/4 -> Resistant moment by FX/13(sin right steer)
  [sinCaster] -> Divide2/2
  Divide2/1 -> [MechanicalTrail]  "Mechanical Trail"
  [MechanicalTrail] -> Total resistance torque by Fy/4(Mechanical Trail)
  Resistant torque by FZ/1(Toral resistance moment by normal force Left) -> [TotalResistanceFzLeft]  "Fz"
  Resistant torque by FZ/2(Toral resistance moment by normal force Right) -> [TotalResistanceFzRight]
  Resistant moment by FX/1(Resistance moment caused by Longitudinal forces left) -> [TotalResistanceFxLeft]  "Fx"
  Resistant moment by FX/2(Resistance moment caused by Longitudinal forces right) -> [TotalResistanceFxRight]
  Total resistance torque by Fy/2(Total resistance moment caused by Fy right) -> [TotalResistanceFyRight]
  Total resistance torque by Fy/1("Total resistance moment caused by FY lefft ") -> [TotalResistanceFyLeft]  "Fy"
  [TotalResistanceFxLeft] -> Tổng lực cản bánh trái/1
  [TotalResistanceFyLeft] -> Tổng lực cản bánh trái/2
  [TotalResistanceFzLeft] -> Tổng lực cản bánh trái/3
  [TotalResistanceFxRight] -> Tổng lực cản bánh phải/1
  [TotalResistanceFyRight] -> Tổng lực cản bánh phải/2
  [TotalResistanceFzRight] -> Tổng lực cản bánh phải/3
  Tổng lực cản bánh trái/1 -> Output of Tổng lực cản bánh trái/1, Tổng lực cản 2 bánh xe/1
  Tổng lực cản bánh phải/1 -> Output of Tổng lực cản bánh phải/1, Tổng lực cản 2 bánh xe/2
  Tổng lực cản 2 bánh xe/1 -> Scope/1, Display/1

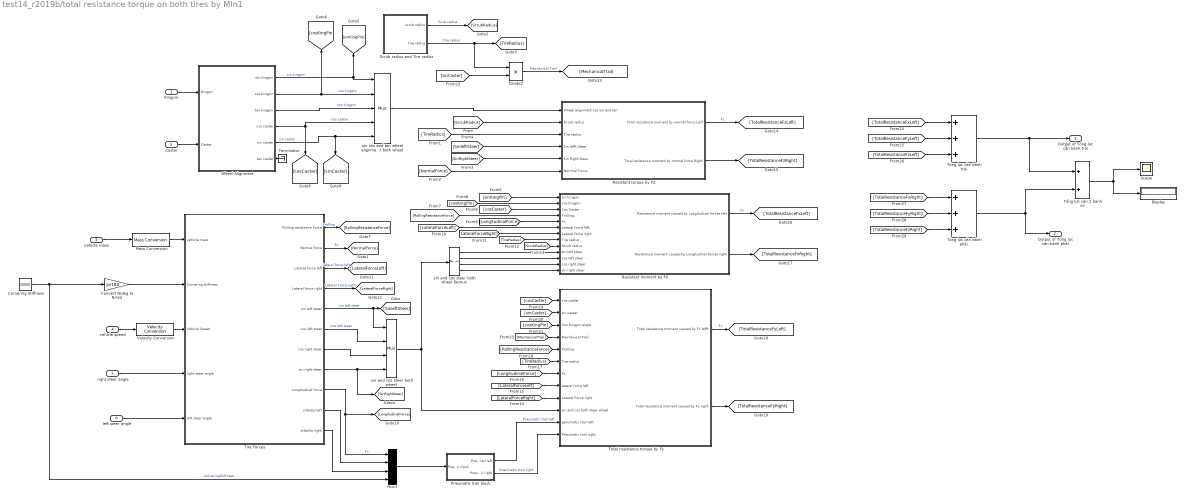
== system test14_r2019b/total resistance torque on both tires by MIn1 ==
  Kingpin : Inport
  Caster : Inport  Port=2
  Vehicle mass : Inport  Port=3
  "vehicle speed " : Inport  Port=4
  right steer angle : Inport  Port=5
  left steer angle : Inport  Port=6
  Convert N/deg to N/rad : Gain  Gain=pi/180
  Cornering Stiffness : Constant  Value=20000
  Display : Display
  Divide2 : Product  Inputs=**
  Mass Conversion : aerolibconvert2/Mass Conversion  IU=kg  OU=kg
  Mux1 : Mux
  Pneumatic trail block : Subsystem
  Resistant moment by FX : Subsystem
  Resistant torque by FZ : Subsystem
  Scope : Scope
  Scrub radius and Tire radius : Subsystem
  Terminator : Terminator
  Tire Forces : Subsystem
  Total resistance torque by Fy : Subsystem
  Tổng lực cản 2 bánh xe : Sum
  Tổng lực cản bánh phải : Sum  Inputs=+++
  Tổng lực cản bánh trái : Sum  Inputs=+++
  Velocity Conversion : aerolibconvert2/Velocity Conversion  IU=km/h  OU=m/s
  Wheel Alignment : Subsystem
  sin and cos steer both wheel : Mux
  sin and cos steer both wheel Demux : Demux
  sin,cos and tan wheel alignment both wheel : Mux  Inputs=5
  Output of Tổng lực cản bánh trái : Outport
  Output of Tổng lực cản bánh phải : Outport  Port=2
  wires:
  Kingpin/1 -> Wheel Alignment/1(Kingpin)
  Wheel Alignment/6(tan caster) -> Terminator/1
  Vehicle mass/1 -> Mass Conversion/1
  Mass Conversion/1 -> Tire Forces/1(vehicle mass)
  Convert N/deg to N/rad/1 -> Tire Forces/2(Cornering stiffness)
  Cornering Stiffness/1 -> Mux1/4, Convert N/deg to N/rad/1  "CorneringStiffness"
  Caster/1 -> Wheel Alignment/2(Caster)
  "vehicle speed "/1 -> Velocity Conversion/1
  right steer angle/1 -> Tire Forces/4("right steer angle ")
  left steer angle/1 -> Tire Forces/5("left steer angle ")
  Velocity Conversion/1 -> Tire Forces/3(Vehicle Speed)
  Tire Forces/11(sideslip right) -> Mux1/3
  Tire Forces/10(sidelsip left) -> Mux1/2
  Tire Forces/9(Longitudinal force) -> [LongitudinalForce], Mux1/1  "Fx"
  Mux1/1 -> Pneumatic trail block/1(Pneumatic trail Input)
  Pneumatic trail block/2(Pneumatic Trail right) -> Total resistance torque by Fy/12(Pneumatic trail right)  "Pneumatic trail right"
  Pneumatic trail block/1(Pneumatic Trail left) -> Total resistance torque by Fy/11(penumatic trail left)  "Pneumatic trail left"
  Tire Forces/5(sin left steer) -> sin and cos steer both wheel/1, [SinleftSteer]  "sin left steer"
  Tire Forces/6(cos left steer) -> sin and cos steer both wheel/2  "cos left steer"
  Tire Forces/7(cos right steer) -> sin and cos steer both wheel/3
  Tire Forces/8(sin right steer) -> [SinRightSteer], sin and cos steer both wheel/4
  sin and cos steer both wheel/1 -> sin and cos steer both wheel Demux/1, Total resistance torque by Fy/10(sin and cos both steer wheel)
  Wheel Alignment/1(sin kingpin) -> sin,cos and tan wheel alignment both wheel/1, [sinKingPin]  "sin kingpin"
  Wheel Alignment/2(cos kingpin) -> [cosKingPin], sin,cos and tan wheel alignment both wheel/2  "cos kingpin"
  Wheel Alignment/3(tan kingpin) -> sin,cos and tan wheel alignment both wheel/3  "tan kingpin"
  Wheel Alignment/4(cos caster) -> sin,cos and tan wheel alignment both wheel/4, [cosCaster]  "cos caster"
  Wheel Alignment/5(sin caster) -> [sinCaster], sin,cos and tan wheel alignment both wheel/5  "sin caster"
  sin,cos and tan wheel alignment both wheel/1 -> Resistant torque by FZ/1("Wheel alignment cos sin and tan ")
  Tire Forces/2(Normal force) -> [NormalForce]  "Fz"
  Scrub radius and Tire radius/1(scrub radius) -> [ScrubRadius]  "Scub radius"
  Scrub radius and Tire radius/2(tire radius) -> Divide2/1, [TireRadius]  "Tire radius"
  [ScrubRadius] -> Resistant torque by FZ/2(Scrub radius)
  [TireRadius] -> Resistant torque by FZ/3(Tire radius)
  [NormalForce] -> Resistant torque by FZ/6(Norrmal Force)
  [SinleftSteer] -> Resistant torque by FZ/4(Sin lefft Steer)
  [SinRightSteer] -> Resistant torque by FZ/5(Sin Right Steer)
  [sinKingPin] -> Resistant moment by FX/1(sin kingpin)
  [cosKingPin] -> Resistant moment by FX/2(cos kingpin)
  Tire Forces/1(Rolling resistance Force) -> [RollingResistanceForce]  "Frolling"
  [RollingResistanceForce] -> Resistant moment by FX/4(Frolling)
  [cosCaster] -> Resistant moment by FX/3(Cos Caster)
  [LongitudinalForce] -> Resistant moment by FX/5(Fx)
  Tire Forces/3(Lateral force left) -> [LateralForceLeft]  "lateral force left"
  Tire Forces/4(Lateral force right) -> [LateralForceRight]  "Lateral Force right"
  [LateralForceLeft] -> Resistant moment by FX/6(Lateral force left)
  [LateralForceRight] -> Resistant moment by FX/7(Lateral force right)
  [TireRadius] -> Resistant moment by FX/8(Tire radius)
  [ScrubRadius] -> Resistant moment by FX/9(Scrub radius)
  [LateralForceRight] -> Total resistance torque by Fy/9(Lateral Force right)
  [LateralForceLeft] -> Total resistance torque by Fy/8(lateral force left)
  [LongitudinalForce] -> Total resistance torque by Fy/7(Fx)
  [TireRadius] -> Total resistance torque by Fy/6(Tire radius)
  [RollingResistanceForce] -> Total resistance torque by Fy/5(Frolling)
  [sinCaster] -> Total resistance torque by Fy/2(sin caster)
  [cosCaster] -> Total resistance torque by Fy/1(cos caster)
  [cosKingPin] -> Total resistance torque by Fy/3(Cos Kingpin angle)
  sin and cos steer both wheel Demux/1 -> Resistant moment by FX/10(sin left steer)
  sin and cos steer both wheel Demux/2 -> Resistant moment by FX/11(cos left steer)
  sin and cos steer both wheel Demux/3 -> Resistant moment by FX/12(cos right steer)
  sin and cos steer both wheel Demux/4 -> Resistant moment by FX/13(sin right steer)
  [sinCaster] -> Divide2/2
  Divide2/1 -> [MechanicalTrail]  "Mechanical Trail"
  [MechanicalTrail] -> Total resistance torque by Fy/4(Mechanical Trail)
  Resistant torque by FZ/1(Toral resistance moment by normal force Left) -> [TotalResistanceFzLeft]  "Fz"
  Resistant torque by FZ/2(Toral resistance moment by normal force Right) -> [TotalResistanceFzRight]
  Resistant moment by FX/1(Resistance moment caused by Longitudinal forces left) -> [TotalResistanceFxLeft]  "Fx"
  Resistant moment by FX/2(Resistance moment caused by Longitudinal forces right) -> [TotalResistanceFxRight]
  Total resistance torque by Fy/2(Total resistance moment caused by Fy right) -> [TotalResistanceFyRight]
  Total resistance torque by Fy/1("Total resistance moment caused by FY lefft ") -> [TotalResistanceFyLeft]  "Fy"
  [TotalResistanceFxLeft] -> Tổng lực cản bánh trái/1
  [TotalResistanceFyLeft] -> Tổng lực cản bánh trái/2
  [TotalResistanceFzLeft] -> Tổng lực cản bánh trái/3
  [TotalResistanceFxRight] -> Tổng lực cản bánh phải/1
  [TotalResistanceFyRight] -> Tổng lực cản bánh phải/2
  [TotalResistanceFzRight] -> Tổng lực cản bánh phải/3
  Tổng lực cản bánh trái/1 -> Output of Tổng lực cản bánh trái/1, Tổng lực cản 2 bánh xe/1
  Tổng lực cản bánh phải/1 -> Output of Tổng lực cản bánh phải/1, Tổng lực cản 2 bánh xe/2
  Tổng lực cản 2 bánh xe/1 -> Scope/1, Display/1

== system test14_r2019b/Steering Dynamics/Chassis + Rack ==
  Add : Sum
  Constant : Constant  Value=2.73
  Gain : Gain  Gain=5.4
  Rack Case + Chassis : Subsystem
  Rack_1_RIGID : Subsystem
  Radians to Degrees : simulink_extras/Transformations/Radians to Degrees
  Target : PMIOPort  Side=Left
  Conn3 : PMIOPort  Port=2  Side=Left
  Conn1 : PMIOPort  Port=3  Side=Left
  F2 : PMIOPort  Port=4  Side=Right
  F3 : PMIOPort  Port=5  Side=Right
  Steering Wheel Angle : Outport
  Steering Wheel Velocity : Outport  Port=2
  wires:
  Rack Case + Chassis/1(Steering Wheel Angle) -> Add/1
  Constant/1 -> Add/2
  Add/1 -> Radians to Degrees/1
  Radians to Degrees/1 -> Gain/1
  Gain/1 -> Steering Wheel Angle/1
  Rack Case + Chassis/2(Steering Wheel Velocity) -> Steering Wheel Velocity/1
  connections:
  Rack_1_RIGID/RConn1 -- Rack Case + Chassis/LConn2
  Rack_1_RIGID/RConn2 -- Rack Case + Chassis/LConn3
  Rack_1_RIGID/RConn4 -- Rack Case + Chassis/LConn5
  Conn3/RConn1 -- Rack Case + Chassis/LConn1
  Target/RConn1 -- Rack_1_RIGID/LConn1
  Rack Case + Chassis/LConn4 -- Rack_1_RIGID/RConn3
  Rack Case + Chassis/LConn7 -- F2/RConn1
  Rack Case + Chassis/LConn6 -- Rack_1_RIGID/RConn5
  Rack Case + Chassis/RConn2 -- F3/RConn1
  Rack Case + Chassis/RConn1 -- Conn1/RConn1

== system test14_r2019b/Steering Dynamics/Rod_2_RIGID ==
  ReferenceFrame : sm_lib/Frames and Transforms/Reference Frame
  Solid : sm_lib/Body Elements/File Solid  ExtGeomFileName=Rod_Default_sldprt.STEP  UnitType=FromFile  ExtGeomFileUnits=m  StepReaderType=HEX  ExportConvexHullGeometry=off  InertiaType=Custom  Mass=smiData.Solid(4).mass  MassUnits=kg  CenterOfMass=smiData.Solid(4).CoM  CenterOfMassUnits=mm  MomentsOfInertia=smiData.Solid(4).MoI  MomentsOfInertiaUnits=kg*mm^2  ProductsOfInertia=smiData.Solid(4).PoI  ProductsOfInertiaUnits=kg*mm^2  BasedOnType=DensityFromFile  Density=1000  DensityUnits=kg/m^3  DoExposeReferenceFrame=on  SerializedFrames=<Frames/>  GraphicType=FromGeometry  MarkerShape=Sphere  MarkerSize=10  GraphicVisPropType=SimpleVisualProperties  GraphicDiffuseColor=smiData.Solid(4).color  GraphicSpecularColor=[0.5 0.5 0.5 1.0]  GraphicAmbientColor=[0.15 0.15 0.15 1.0]  GraphicEmissiveColor=[0.0 0.0 0.0 1.0]  GraphicShininess=75  GraphicOpacity=smiData.Solid(4).opacity
  Transform : sm_lib/Frames and Transforms/Rigid Transform  TranslationMethod=Cartesian  TranslationStandardOffset=0  TranslationLengthUnit=mm  TranslationStandardAxis=+Z  TranslationCartesianOffset=smiData.RigidTransform(39).translation  TranslationROffset=0  TranslationROffsetUnits=m  TranslationZOffset=0  TranslationZOffsetUnits=m  TranslationThetaOffset=0  TranslationThetaOffsetUnits=deg  RotationMethod=ArbitraryAxis  RotationAngleUnits=rad  RotationStandardAxis=+Z  RotationAngle=smiData.RigidTransform(39).angle  RotationArbitraryAxis=smiData.RigidTransform(39).axis  FollAlignAxisA=+X  BaseAlignAxisA=+Y  FollAlignAxisB=+Y  BaseAlignAxisB=+Z  RotationSequenceAxes=FollowerAxes  RotationSequence=XYX  RotationSequenceAngles=[0 0 0]  RotationSequenceAnglesUnits=deg  RotationMatrix=[1 0 0; 0 1 0; 0 0 1]  Quaternion=[1 0 0 0]
  Transform1 : sm_lib/Frames and Transforms/Rigid Transform  TranslationMethod=Cartesian  TranslationStandardOffset=0  TranslationLengthUnit=mm  TranslationStandardAxis=+Z  TranslationCartesianOffset=smiData.RigidTransform(42).translation  TranslationROffset=0  TranslationROffsetUnits=m  TranslationZOffset=0  TranslationZOffsetUnits=m  TranslationThetaOffset=0  TranslationThetaOffsetUnits=deg  RotationMethod=ArbitraryAxis  RotationAngleUnits=rad  RotationStandardAxis=+Z  RotationAngle=smiData.RigidTransform(42).angle  RotationArbitraryAxis=smiData.RigidTransform(42).axis  FollAlignAxisA=+X  BaseAlignAxisA=+Y  FollAlignAxisB=+Y  BaseAlignAxisB=+Z  RotationSequenceAxes=FollowerAxes  RotationSequence=XYX  RotationSequenceAngles=[0 0 0]  RotationSequenceAnglesUnits=deg  RotationMatrix=[1 0 0; 0 1 0; 0 0 1]  Quaternion=[1 0 0 0]
  F : PMIOPort  Side=Left
  F1 : PMIOPort  Port=2  Side=Right
  connections:
  Solid/RConn1 -- ReferenceFrame/RConn1 -- Transform/LConn1 -- Transform1/LConn1
  Transform/RConn1 -- F/RConn1
  Transform1/RConn1 -- F1/RConn1

== system test14_r2019b/Steering Dynamics/Sensing  ==
  Add : Sum
  Add1 : Sum
  Constant1 : Constant  Value=1.5458-2.6414e-05+0.01940853136
  Constant2 : Constant  Value=1.5847-(-2.3866e-05)-0.019541748665
  Gain1 : Gain  Gain=-1
  PS-Simulink Converter : nesl_utility/PS-Simulink Converter  PhysicalDomain=network_engine_domain  SubClassName=ps_output  LeftPortType=input  RightPortType=output  PseudoPeriodic=off  Frequencies=[]  VectorFormat=1-D array  Unit=rad  AffineConversion=off
  PS-Simulink Converter1 : nesl_utility/PS-Simulink Converter  PhysicalDomain=network_engine_domain  SubClassName=ps_output  LeftPortType=input  RightPortType=output  PseudoPeriodic=off  Frequencies=[]  VectorFormat=1-D array  Unit=rad  AffineConversion=off
  Radians to Degrees : simulink_extras/Transformations/Radians to Degrees
  Radians to Degrees1 : simulink_extras/Transformations/Radians to Degrees
  Scope : Scope  NumInputPorts=2
  To Workspace : ToWorkspace  VariableName=left  SaveFormat=Structure  SampleTime=-1
  To Workspace1 : ToWorkspace  VariableName=right  SaveFormat=Structure  SampleTime=-1
  for left : MATLAB Function  TreatAsAtomicUnit=on
  for right : MATLAB Function  TreatAsAtomicUnit=on
  input : PMIOPort  Side=Left
  input1 : PMIOPort  Port=2  Side=Left
  Steering angle left (rad) : Outport
  Steering angle right (rad) : Outport  Port=2
  wires:
  Constant1/1 -> Add/2
  PS-Simulink Converter1/1 -> Radians to Degrees1/1, Add1/1, To Workspace1/1  "Steering angle right (rad)"
  PS-Simulink Converter/1 -> To Workspace/1, Radians to Degrees/1, Add/1  "Steering angle left (rad)"
  Constant2/1 -> Add1/2
  Add/1 -> for left/1(input)  "Steering angle left (rad)"
  Add1/1 -> Gain1/1  "Steering angle right (rad)"
  Radians to Degrees/1 -> Scope/1  "left"
  Radians to Degrees1/1 -> Scope/2  "right"
  Gain1/1 -> for right/1(input)
  for left/1(output) -> Steering angle left (rad)/1
  for right/1(output) -> Steering angle right (rad)/1
  connections:
  input/RConn1 -- PS-Simulink Converter/LConn1
  input1/RConn1 -- PS-Simulink Converter1/LConn1
